simulink model "test1"  (R2023a)
settings: Solver=VariableStepAuto  StartTime=0.0  StopTime=40  MaxStep=1e-6  RelTol=1e-3
values from neighbouring files (symbols this model uses):
  Ce = 0.1459    [test.m]
  R = 0.368    [test.m]
  Tl = 0.0144    [test.m]
  Tm = 0.18    [test.m]
libraries: spsDCVoltageSourceLib x1, slpidlib x1, simulink x1, spsUniversalBridgeLib x1, spsVoltageMeasurementLib x1, spspowerguiLib x1
settings Model: Creator=LENOVO  LastModifiedBy=LENOVO

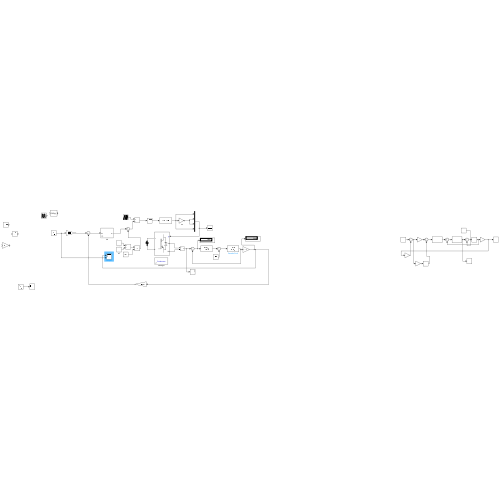
[thumbnail: Simulink's stored preview of the top-level diagram]
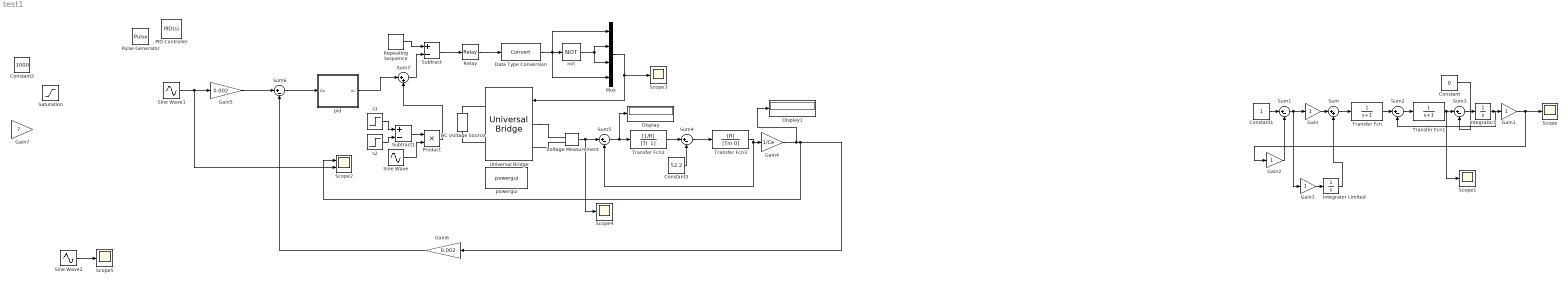
== system test1 ==
  Constant : Constant  Value=0
  Constant1 : Constant
  Constant2 : Constant  Value=1000
  Constant3 : Constant  Value=52.2
  DC Voltage Source : spsDCVoltageSourceLib/DC Voltage Source  Amplitude=538  Measurements=None
  Data Type Conversion : DataTypeConversion  SaturateOnIntegerOverflow=off  RndMeth=Floor
  Display : Display
  Display1 : Display
  Gain{,1..3} (4 alike) : Gain
  Gain4 : Gain  Gain=1/Ce
  Gain5 : Gain  Gain=0.002
  Gain6 : Gain  Gain=0.002
  Gain7 : Gain  Gain=7
  Integrator Limited : Integrator  LimitOutput=on  UpperSaturationLimit=10  LowerSaturationLimit=-10
  Integrator1 : Integrator
  Mux : Mux
  PID Controller : slpidlib/PID Controller  Controller=PID  Form=Parallel  TimeDomain=Continuous-time  UseExternalTs=off  SampleTime=-1  IntegratorMethod=Forward Euler  FilterMethod=Forward Euler  ControllerParametersSource=internal  P=1  I=1  UseKiTs=off  D=0  N=100  UseFilter=on  TunerSelectOption=Transfer Function Based (PID Tuner App)  InitialConditionSource=internal  InitialConditionForIntegrator=0  InitialConditionForFilter=0  DifferentiatorICPrevScaledInput=0  ExternalReset=none  TrackingMode=off  Kt=1  LimitOutput=off  SatLimitsSource=internal  UpperSaturationLimit=inf  LowerSaturationLimit=-inf  LinearizeAsGain=on  AntiWindupMode=none  Kb=1  LimitIntegrator=off  UpperIntegratorSaturationLimit=inf  LowerIntegratorSaturationLimit=-inf  POutMin=[]  POutMax=[]  IOutMin=[]  IOutMax=[]  DOutMin=[]  DOutMax=[]  NOutMin=[]  NOutMax=[]  SumOutMin=[]  SumOutMax=[]  SaturationOutMin=[]  SaturationOutMax=[]  PParamMin=[]  PParamMax=[]  IParamMin=[]  IParamMax=[]  DParamMin=[]  DParamMax=[]  NParamMin=[]  NParamMax=[]  KbParamMin=[]  KbParamMax=[]  KtParamMin=[]  KtParamMax=[]  KbOutMin=[]  KbOutMax=[]  KtOutMin=[]  KtOutMax=[]  IntegratorOutMin=[]  IntegratorOutMax=[]  FilterOutMin=[]  FilterOutMax=[]  SumI1OutMin=[]  SumI1OutMax=[]  SumI2OutMin=[]  SumI2OutMax=[]  SumI3OutMin=[]  SumI3OutMax=[]  SumI4OutMin=[]  SumI4OutMax=[]  SumDOutMin=[]  SumDOutMax=[]  DifferentiatorOutMin=[]  DifferentiatorOutMax=[]  FilterDiffOutCoefMin=[]  FilterDiffOutCoefMax=[]  ReciprocalOutMin=[]  ReciprocalOutMax=[]  SumDenOutMin=[]  SumDenOutMax=[]  SumNumOutMin=[]  SumNumOutMax=[]  DivideOutMin=[]  DivideOutMax=[]  UdiffTsProdOutMin=[]  UdiffTsProdOutMax=[]  NTsProdOutMin=[]  NTsProdOutMax=[]  UintegralTsProdOutMin=[]  UintegralTsProdOutMax=[]  UngainTsProdOutMin=[]  UngainTsProdOutMax=[]  ClampingZeroOutDataTypeStr=Inherit: Inherit via back propagation  ClampingZeroOutMin=[]  ClampingZeroOutMax=[]  FilterDenConstantOutDataTypeStr=Inherit: Inherit via back propagation  FilterDenConstantOutMin=[]  FilterDenConstantOutMax=[]  PCopyOutDataTypeStr=Inherit: Inherit via back propagation  PCopyOutMin=[]  PCopyOutMax=[]  NCopyOutDataTypeStr=Inherit: Inherit via back propagation  NCopyOutMin=[]  NCopyOutMax=[]  IntegratorContinuousStateAttributes=''  IntegratorStateMustResolveToSignalObject=off  IntegratorRTWStateStorageClass=Auto  FilterContinuousStateAttributes=''  FilterStateMustResolveToSignalObject=off  FilterRTWStateStorageClass=Auto  ParallelPVariant=InternalParameters  IdealPVariant=Disabled  IVariant=InternalParameters  DVariant=InternalParameters  IntegratorVariant=Continuous  SatVariant=Disabled  AWVariant=Passthrough  PCopyVariant=Disabled  TRVariant=Disabled  FdbkBlocksVariant=Forward  IdealPFdbkVariant=Disabled  SatFdbkVariant=Disabled  DerivativeFilterVariant=ContFilter  NVariant=InternalParameters  NCopyVariant=Disabled  FilterICVariant=InternalICsFilter  IntegratorICVariant=InternalICs  ExternalResetVariant=Disabled  TRSumVariant=Passthrough  SumFdbkVariant=Disabled  SumVariant=Sum_PID  TsampFilterVariant=InternalTs  TsampNgainVariant=Passthrough  TsampIntegralVariant=Disabled_SignalSpec  ExternalSaturationOutDataTypeStr=Inherit: Same as second input
  Product : Product
  Pulse Generator : DiscretePulseGenerator  PulseType=Time based  Period=1/8000  PulseWidth=400/538/2*100+50
  Relay : Relay  OnOutputValue=0  OffOutputValue=1
  Repeating Sequence : simulink/Sources/Repeating Sequence  rep_seq_t=[0 1/8000]  rep_seq_y=[-5 5]
  Saturation : Saturate  UpperLimit=5  LowerLimit=-5
  Scope{,1,3..5} (5 alike) : Scope
  Scope2 : Scope  NumInputPorts=2
  Sine Wave : Sin  Amplitude=0.5  Frequency=pi  SampleTime=0
  Sine Wave1 : Sin  Amplitude=1000  SampleTime=0
  Sine Wave2 : Sin  Amplitude=1000  SampleTime=0
  Subtract : Sum  Inputs=+-
  Subtract1 : Sum  Inputs=+-
  Sum : Sum  Inputs=|++
  Sum{1..6} (6 alike) : Sum  Inputs=|+-
  Sum7 : Sum  Inputs=|++
  Transfer Fcn : TransferFcn  Denominator=[1 1]
  Transfer Fcn1 : TransferFcn  Denominator=[1 1]
  Transfer Fcn2 : TransferFcn  Numerator=[1/R]  Denominator="[Tl  1]"
  Transfer Fcn3 : TransferFcn  Numerator=[R]  Denominator=[Tm 0]
  Universal Bridge : spsUniversalBridgeLib/Universal Bridge  Arms=2  SnubberResistance=1e5  SnubberCapacitance=inf  Device=IGBT / Diodes  Ron=1e-3  Lon=0  ForwardVoltages="[  0  0]"  ForwardVoltage=0  GTOparameters=[ 10e-6 , 20e-6 ]  IGBTparameters=[ 1e-6 , 2e-6 ]  Measurements=None  Measurements_2=None  converterType=Rectifier
  Voltage Measurement : spsVoltageMeasurementLib/Voltage Measurement  PhasorSimulation=off  OutputType=Complex  PSBequivalent=0
  not : Logic  Operator=NOT  IconShape=distinctive  AllPortsSameDT=off  OutDataTypeStr=boolean
  pid : Subsystem  mask{kp=7, ki=10}
      mask DialogControl ParameterGroupVar Prompt: 参数
  powergui : spspowerguiLib/powergui  Priority=1  SimulationMode=Continuous  SampleTime=50e-6  frequency=60  Iterations=50  frequencyindice=0  Pbase=100e6  ErrMax=1e-4  UnitsV=kV  UnitsW=MW  buscounter=0  FunctionMessages=off  echomessages=off  EnableUseOfTLC=off  CurrentSourceSwitches=off  DisableSnubberDevices=off  DisableRonSwitches=off  DisableVfSwitches=off  DisplayEquations=off  AutomaticDiscreteSolvers=off  SolverType=Tustin/Backward Euler (TBE)  Interpol=off  ExternalGateDelay=off  methode=off  Ts=100  x0status=blocks  SPID=on  SwTol=0  HookPort=off  NonlinearTolerance=1e-4  nMaxIteration=100  ContinueOnMaxIteration=off  RestoreLinks=warning  ResistiveCurrentMeasurement=off  Frange=[0:2:500]  Ylog=off  Xlog=on  ShowGrid=off  save=off  variable=ZData  structure=0  ZoomFFT=off  StartTime=0.0  cycles=1  DisplayStyle=1  fundamental=60  FreqAxis=off  MaxFrequency=1000  frequencyindicesteady=1  RmsSteady=1  display=off
  s1 : Step  Time=20  SampleTime=0
  s2 : Step  Time=30  SampleTime=0
  wires:
  Gain/1 -> Sum/1
  Integrator Limited/1 -> Sum/2
  Sum1/1 -> Gain/1, Gain3/1
  Sum/1 -> Transfer Fcn/1
  Transfer Fcn/1 -> Sum2/1
  Sum2/1 -> Transfer Fcn1/1
  Transfer Fcn1/1 -> Scope1/1, Sum3/1
  Sum3/1 -> Integrator1/1
  Integrator1/1 -> Sum2/2, Gain1/1
  Constant/1 -> Sum3/2
  Constant1/1 -> Sum1/1
  Gain1/1 -> Gain2/1, Scope/1
  Gain2/1 -> Sum1/2
  Gain3/1 -> Integrator Limited/1
  Voltage Measurement/1 -> Scope4/1, Sum5/1
  Constant3/1 -> Sum4/2
  Transfer Fcn2/1 -> Sum4/1
  Gain4/1 -> Scope2/1, Gain6/1, Display1/1
  Sum4/1 -> Transfer Fcn3/1
  Sum5/1 -> Display/1, Transfer Fcn2/1
  Transfer Fcn3/1 -> Sum5/2, Gain4/1
  Data Type Conversion/1 -> Mux/4, Mux/1, not/1
  not/1 -> Mux/3, Mux/2
  Mux/1 -> Scope3/1, Universal Bridge/1
  Repeating Sequence/1 -> Subtract/1
  Subtract/1 -> Relay/1
  Relay/1 -> Data Type Conversion/1
  Sum6/1 -> pid/1(du)
  Gain5/1 -> Sum6/1
  Gain6/1 -> Sum6/2
  pid/1(uc) -> Sum7/1
  Sum7/1 -> Subtract/2
  Sine Wave1/1 -> Scope2/2, Gain5/1
  Product/1 -> Sum7/2
  Sine Wave/1 -> Product/2
  s2/1 -> Subtract1/2
  Subtract1/1 -> Product/1
  s1/1 -> Subtract1/1
  Sine Wave2/1 -> Scope5/1
  connections:
  DC Voltage Source/RConn1 -- Universal Bridge/RConn1
  DC Voltage Source/LConn1 -- Universal Bridge/RConn2
  Universal Bridge/LConn1 -- Voltage Measurement/LConn1
  Voltage Measurement/LConn2 -- Universal Bridge/LConn2

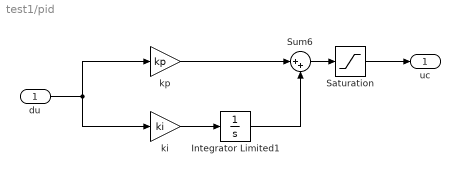
== system test1/pid ==
  du : Inport
  Integrator Limited1 : Integrator  LimitOutput=on  UpperSaturationLimit=5  LowerSaturationLimit=-5
  Saturation : Saturate  UpperLimit=5  LowerLimit=-5
  Sum6 : Sum  Inputs=|++
  ki : Gain  Gain=ki
  kp : Gain  Gain=kp
  uc : Outport
  wires:
  du/1 -> kp/1, ki/1
  ki/1 -> Integrator Limited1/1
  Integrator Limited1/1 -> Sum6/2
  kp/1 -> Sum6/1
  Sum6/1 -> Saturation/1
  Saturation/1 -> uc/1
